simulink model "sampleModel1640"  (R2023a)
settings: Solver=VariableStepAuto  StartTime=0.0  StopTime=10.0  RelTol=1e-3
libraries: hdlsllib x5, simulink x2
settings Model: Creator=user1  LastModifiedBy=user1

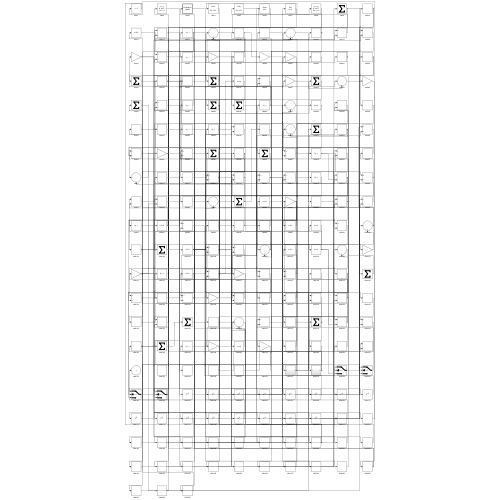
[thumbnail: Simulink's stored preview of the top-level diagram]
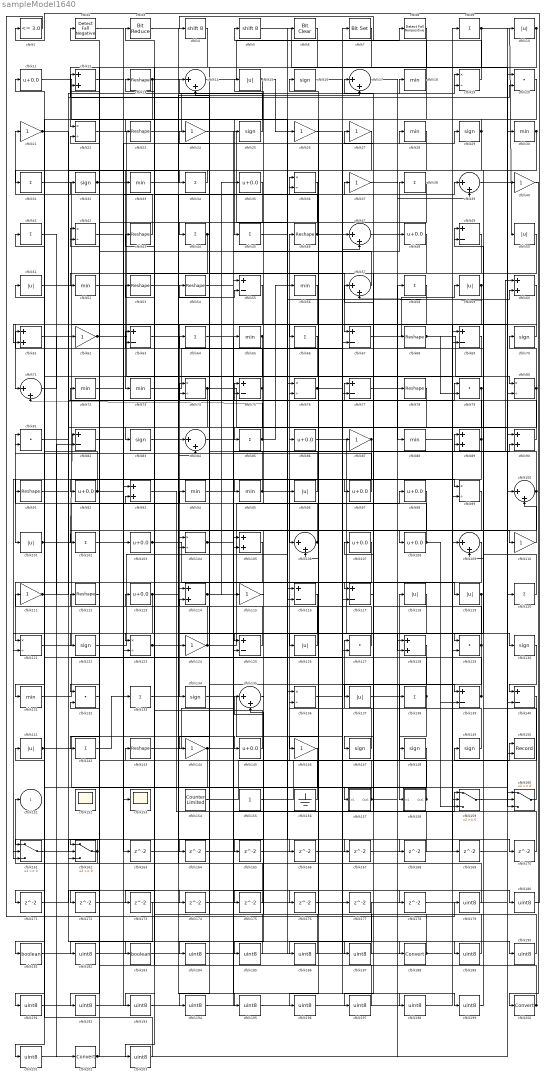
== system sampleModel1640 ==
  cfblk1 : hdlsllib/Logic and Bit Operations/Compare To Constant  relop=<=  const=3.0  OutDataTypeStr=boolean
  cfblk{10,15,50..51,59,96,101,118..119,126,137,141} (12 alike) : Abs  SaturateOnIntegerOverflow=off
  cfblk{14,17,39,47,57,71,84,100,106,109,135} (11 alike) : Sum  Inputs=|++
  cfblk{9,31,34,38,41,44..45,58,64,66,85,102,120,133,138,142} (16 alike) : Sum  Inputs=+
  cfblk{11,35,48,86,92,97..98,103,107..108,113,145} (12 alike) : Bias  Bias=0.0  SaturateOnIntegerOverflow=off
  cfblk{19,22,36,42,74,76,80,99,104,121,123,136} (12 alike) : Product  Inputs=*/  RndMeth=Zero  SaturateOnIntegerOverflow=on
  cfblk{12,60..61,89..90,93,105,114,128} (9 alike) : Sum
  cfblk{21,24,26..27,37,40,62,87,110..111,115,124,144,146} (14 alike) : Gain
  cfblk{13,23,43,46,53..54,68,78,91,112,143} (11 alike) : Reshape
  cfblk{49,55,63,67,69,75,77,82,116..117,125,139..140} (13 alike) : Sum  Inputs=+-
  cfblk{16,25,29,32,70,83,122,130,134,147..149} (12 alike) : Signum
  cfblk{20,79,81,127,129,132} (6 alike) : DotProduct  OutDataTypeStr=Inherit: Inherit via internal rule
  cfblk{18,28,30,33,52,56,65,72..73,88,94..95,131} (13 alike) : MinMax
  cfblk150 : Record  FileSettingsInternal="{\"entries\":[{\"content\":{\"excelSettings\":{\"content\":{},\"type\":\"Streamout.ExcelSettings\"}},\"type\":\"Streamout.FileSettingStorage\",\"uuid\":\"\"}],\"packageUris\":[\"http:\\/\\/schema.mathworks.com\\/mf0\\/streamout_blocks\\/R2020a\"],\"version\":\"1.0\"}"  Layout=[1 1]  SignalsInternal="{\"entries\":[{\"content\":{\"signals\":[{\"content\":{\"blockPath\":[],\"dimensions\":[1],\"domain\":\"\",\"lineColor\":\"#a2142f\",\"plots\":[1],\"port\":1,\"sid\":[\"\"],\"signalID\":2475,\"signalName\":\"cfblk157\"},\"type\":\"RecordBlkView.Signal\",\"uuid\":\"\"},{\"content\":{\"blockPath\":[],\"dimensions\":[1],\"domain\":\"\",\"lineColor\":\"#139fff\",\"plots\":[1],\"port\":2,\"sid\":[\"\"],\"signalID\":2479,\"signalName\":\"cfblk10\"},\"type\":\"RecordBlkView.Signal\",\"uuid\":\"\"}]},\"type\":\"RecordBlkView.InputSignals\",\"uuid\":\"\"}],\"packageUris\":[\"http:\\/\\/schema.mathworks.com\\/mf0\\/streamout_blocks\\/R2020a\"],\"version\":\"1.0\"}"  VisualizationBindings="{\"xyplotplugin\":{\"info\":[{\"series\":[{\"bindingParametersList\":[{\"parameter\":\"X-Axis\",\"signalID\":2475,\"signalName\":\"cfblk157\"},{\"parameter\":\"Y-Axis\",\"signalID\":2479,\"signalName\":\"cfblk10\"}],\"seriesID\":51744}],\"subplotID\":1}]}}"  CompatibilityTag=XY  st=-1
  cfblk152 : Scope
      settings: Floating=on
  cfblk153 : Scope
  cfblk154 : hdlsllib/Sources/Counter Limited  uplimit=7  tsamp=-1
  cfblk155 : Constant  SampleTime=-1
  cfblk156 : Ground
  cfblk157 : Subsystem
      settings: LibrarySourceBlock=|
      | hdlsllib/Ports &
      | Subsystems/Subsystem
  cfblk158 : Subsystem
      settings: LibrarySourceBlock=|
      | hdlsllib/Ports &
      | Subsystems/Subsystem
  cfblk{159..162} (4 alike) : Switch  SaturateOnIntegerOverflow=off  InputSameDT=off
  cfblk{163..178} (16 alike) : Delay  SampleTime=1
  cfblk{179..180,182,184..187,189..199,201,203} (20 alike) : DataTypeConversion  OutDataTypeStr=uint8  SaturateOnIntegerOverflow=off  RndMeth=Floor
  cfblk181 : DataTypeConversion  OutDataTypeStr=boolean  SaturateOnIntegerOverflow=off  RndMeth=Floor
  cfblk183 : DataTypeConversion  OutDataTypeStr=boolean  SaturateOnIntegerOverflow=off  RndMeth=Floor
  cfblk188 : DataTypeConversion  SaturateOnIntegerOverflow=off  RndMeth=Floor
  cfblk2 : hdlsllib/Logic and Bit Operations/Detect Fall Negative  vinit=0  OutDataTypeStr=boolean
  cfblk200 : DataTypeConversion  SaturateOnIntegerOverflow=off  RndMeth=Floor
  cfblk202 : DataTypeConversion  SaturateOnIntegerOverflow=off  RndMeth=Floor
  cfblk3 : hdlsllib/Logic and Bit Operations/Bit Reduce  mode=AND
  cfblk4 : ArithShift  BitShiftNumber=8
  cfblk5 : ArithShift  BitShiftNumber=8
  cfblk6 : simulink/Logic and Bit Operations/Bit Clear  iBit=0
      settings: LibrarySourceBlock=|
      | hdlsllib/Logic and Bit
      | Operations/Bit Clear
  cfblk7 : simulink/Logic and Bit Operations/Bit Set  iBit=0
      settings: LibrarySourceBlock=|
      | hdlsllib/Logic and Bit
      | Operations/Bit Set
  cfblk8 : hdlsllib/Logic and Bit Operations/Detect Fall Nonpositive  vinit=0  OutDataTypeStr=boolean
  cfblk151 : Outport  VectorParamsAs1DForOutWhenUnconnected=off
  wires:
  cfblk35/1 -> cfblk44/1
  cfblk58/1 -> cfblk134/1
  cfblk86/1 -> cfblk130/1
  cfblk114/1 -> cfblk98/1, cfblk117/1, cfblk35/1
  cfblk31/1 -> cfblk95/1
  cfblk4/1 -> cfblk22/1
  cfblk120/1 -> cfblk64/1
  cfblk97/1 -> cfblk81/1
  cfblk156/1 -> cfblk46/1
  cfblk132/1 -> cfblk12/1
  cfblk41/1 -> cfblk202/1
  cfblk93/1 -> cfblk159/1
  cfblk27/1 -> cfblk73/1
  cfblk149/1 -> cfblk127/1
  cfblk89/1 -> cfblk106/1, cfblk42/2
  cfblk140/1 -> cfblk149/1
  cfblk94/1 -> cfblk89/1
  cfblk144/1 -> cfblk48/1, cfblk173/1
  cfblk65/1 -> cfblk74/2, cfblk181/1
  cfblk101/1 -> cfblk82/1, cfblk20/2
  cfblk130/1 -> cfblk140/1
  cfblk49/1 -> cfblk137/1
  cfblk19/1 -> cfblk4/1
  cfblk98/1 -> cfblk126/1
  cfblk17/1 -> cfblk88/1
  cfblk71/1 -> cfblk62/1
  cfblk147/1 -> cfblk16/1
  cfblk107/1 -> cfblk121/1
  cfblk47/1 -> cfblk38/1
  cfblk80/1 -> cfblk70/1, cfblk203/1
  cfblk139/1 -> cfblk111/1, cfblk138/1
  cfblk100/1 -> cfblk60/1, cfblk36/1, cfblk142/1
  cfblk38/1 -> cfblk92/1
  cfblk119/1 -> cfblk157/1(In1), cfblk125/2
  cfblk56/1 -> cfblk71/1
  cfblk15/1 -> cfblk45/1, cfblk26/1
  cfblk32/1 -> cfblk116/1, cfblk36/2
  cfblk121/1 -> cfblk94/1
  cfblk66/1 -> cfblk114/1
  cfblk9/1 -> cfblk50/1, cfblk123/2
  cfblk18/1 -> cfblk5/1, cfblk196/1
  cfblk87/1 -> cfblk101/1, cfblk117/2, cfblk161/3
  cfblk14/1 -> cfblk8/1
  cfblk110/1 -> cfblk100/2
  cfblk137/1 -> cfblk158/1(In1)
  cfblk124/1 -> cfblk76/1, cfblk93/2
  cfblk48/1 -> cfblk124/1
  cfblk154/1 -> cfblk118/1
  cfblk123/1 -> cfblk39/1, cfblk43/1
  cfblk28/1 -> cfblk131/1
  cfblk142/1 -> cfblk133/1
  cfblk70/1 -> cfblk66/1
  cfblk43/1 -> cfblk21/1
  cfblk145/1 -> cfblk53/1
  cfblk22/1 -> cfblk67/1
  cfblk104/1 -> cfblk65/1, cfblk24/1, cfblk198/1
  cfblk50/1 -> cfblk147/1
  cfblk25/1 -> cfblk14/1
  cfblk73/1 -> cfblk47/1
  cfblk160/1 -> cfblk49/1
  cfblk52/1 -> cfblk33/1
  cfblk85/1 -> cfblk71/2, cfblk56/1
  cfblk37/1 -> cfblk39/2
  cfblk106/1 -> cfblk86/1, cfblk15/1
  cfblk3/1 -> cfblk84/1
  cfblk112/1 -> cfblk72/1
  cfblk141/1 -> cfblk145/1, cfblk160/3
  cfblk68/1 -> cfblk80/1, cfblk79/2
  cfblk157/1(Out1) -> cfblk150/1, cfblk90/2, cfblk76/2
  cfblk75/1 -> cfblk61/1, cfblk132/1
  cfblk23/1 -> cfblk19/1
  cfblk60/1 -> cfblk159/2
  cfblk51/1 -> cfblk120/1
  cfblk159/1 -> cfblk30/1
  cfblk125/1 -> cfblk112/1
  cfblk67/1 -> cfblk59/1
  cfblk79/1 -> cfblk85/1, cfblk102/1
  cfblk20/1 -> cfblk106/2
  cfblk126/1 -> cfblk74/1
  cfblk46/1 -> cfblk108/1, cfblk3/1
  cfblk158/1(Out1) -> cfblk63/1, cfblk42/1
  cfblk29/1 -> cfblk23/1, cfblk67/2
  cfblk34/1 -> cfblk31/1
  cfblk24/1 -> cfblk96/1
  cfblk127/1 -> cfblk11/1
  cfblk62/1 -> cfblk162/1, cfblk99/2
  cfblk55/1 -> cfblk61/2
  cfblk92/1 -> cfblk51/1, cfblk28/1
  cfblk63/1 -> cfblk55/2
  cfblk90/1 -> cfblk77/1
  cfblk136/1 -> cfblk188/1
  cfblk102/1 -> cfblk37/1
  cfblk5/1 -> cfblk140/2
  cfblk11/1 -> cfblk116/2
  cfblk95/1 -> cfblk60/2, cfblk12/2
  cfblk13/1 -> cfblk52/1, cfblk84/2, cfblk91/1
  cfblk21/1 -> cfblk34/1, cfblk176/1
  cfblk122/1 -> cfblk89/2
  cfblk117/1 -> cfblk17/1
  cfblk59/1 -> cfblk97/1, cfblk57/2
  cfblk81/1 -> cfblk18/1
  cfblk103/1 -> cfblk119/1, cfblk110/1, cfblk128/2, cfblk75/1, cfblk75/2
  cfblk16/1 -> cfblk19/2
  cfblk39/1 -> cfblk10/1
  cfblk36/1 -> cfblk123/1
  cfblk162/1 -> cfblk151/1, cfblk161/1
  cfblk57/1 -> cfblk2/1
  cfblk40/1 -> cfblk200/1
  cfblk33/1 -> cfblk17/2
  cfblk138/1 -> cfblk148/1, cfblk32/1
  cfblk143/1 -> cfblk25/1
  cfblk113/1 -> cfblk104/2, cfblk161/2
  cfblk30/1 -> cfblk129/1, cfblk162/2
  cfblk8/1 -> cfblk122/1
  cfblk77/1 -> cfblk68/1
  cfblk64/1 -> cfblk115/1
  cfblk54/1 -> cfblk29/1
  cfblk76/1 -> cfblk139/1, cfblk199/1
  cfblk155/1 -> cfblk129/2
  cfblk42/1 -> cfblk153/1
  cfblk10/1 -> cfblk83/1, cfblk150/2
  cfblk108/1 -> cfblk81/2, cfblk159/3, cfblk139/2
  cfblk118/1 -> cfblk121/2
  cfblk74/1 -> cfblk160/2, cfblk162/3
  cfblk116/1 -> cfblk125/1
  cfblk131/1 -> cfblk87/1
  cfblk111/1 -> cfblk79/1, cfblk82/2, cfblk174/1
  cfblk2/1 -> cfblk93/1
  cfblk96/1 -> cfblk14/2
  cfblk44/1 -> cfblk144/1, cfblk172/1
  cfblk12/1 -> cfblk99/1
  cfblk129/1 -> cfblk27/1, cfblk146/1, cfblk107/1
  cfblk72/1 -> cfblk163/1
  cfblk163/1 -> cfblk127/2
  cfblk128/1 -> cfblk164/1
  cfblk164/1 -> cfblk77/2
  cfblk115/1 -> cfblk165/1
  cfblk165/1 -> cfblk160/1
  cfblk82/1 -> cfblk166/1
  cfblk166/1 -> cfblk47/2
  cfblk45/1 -> cfblk167/1
  cfblk167/1 -> cfblk20/1
  cfblk26/1 -> cfblk168/1
  cfblk168/1 -> cfblk57/1
  cfblk88/1 -> cfblk169/1
  cfblk169/1 -> cfblk49/2
  cfblk161/1 -> cfblk170/1
  cfblk170/1 -> cfblk55/1
  cfblk146/1 -> cfblk171/1
  cfblk172/1 -> cfblk90/1
  cfblk174/1 -> cfblk114/2
  cfblk99/1 -> cfblk175/1
  cfblk175/1 -> cfblk104/1
  cfblk176/1 -> cfblk80/2
  cfblk134/1 -> cfblk177/1
  cfblk133/1 -> cfblk178/1
  cfblk178/1 -> cfblk100/1
  cfblk1/1 -> cfblk179/1
  cfblk179/1 -> cfblk141/1
  cfblk171/1 -> cfblk180/1
  cfblk180/1 -> cfblk1/1
  cfblk181/1 -> cfblk7/1
  cfblk7/1 -> cfblk182/1
  cfblk182/1 -> cfblk78/1
  cfblk91/1 -> cfblk183/1
  cfblk183/1 -> cfblk6/1
  cfblk6/1 -> cfblk184/1
  cfblk184/1 -> cfblk9/1
  cfblk135/1 -> cfblk185/1
  cfblk185/1 -> cfblk113/1
  cfblk177/1 -> cfblk186/1
  cfblk186/1 -> cfblk135/1
  cfblk53/1 -> cfblk187/1
  cfblk187/1 -> cfblk135/2
  cfblk188/1 -> cfblk143/1, cfblk54/1
  cfblk61/1 -> cfblk189/1
  cfblk189/1 -> cfblk136/1
  cfblk84/1 -> cfblk190/1
  cfblk190/1 -> cfblk136/2
  cfblk105/1 -> cfblk191/1
  cfblk191/1 -> cfblk103/1
  cfblk173/1 -> cfblk192/1
  cfblk192/1 -> cfblk105/1
  cfblk78/1 -> cfblk193/1
  cfblk193/1 -> cfblk105/2
  cfblk69/1 -> cfblk194/1
  cfblk194/1 -> cfblk128/1
  cfblk83/1 -> cfblk195/1
  cfblk195/1 -> cfblk69/1
  cfblk196/1 -> cfblk69/2
  cfblk109/1 -> cfblk197/1
  cfblk197/1 -> cfblk22/2
  cfblk198/1 -> cfblk109/1
  cfblk199/1 -> cfblk109/2
  cfblk200/1 -> cfblk63/2, cfblk13/1
  cfblk148/1 -> cfblk201/1
  cfblk201/1 -> cfblk40/1
  cfblk202/1 -> cfblk132/2, cfblk58/1
  cfblk203/1 -> cfblk41/1

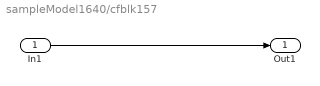
== system sampleModel1640/cfblk157 ==
  In1 : Inport
  Out1 : Outport
  wires:
  In1/1 -> Out1/1

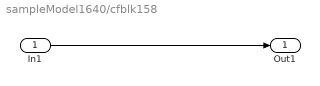
== system sampleModel1640/cfblk158 ==
  In1 : Inport
  Out1 : Outport
  wires:
  In1/1 -> Out1/1
